simulink model "cic_dec3_poly_model"  (Simulink 7.4)
settings: Solver=ode45  StartTime=0.0  StopTime=10.0  RelTol=1e-3
libraries: xbsIndex_r4 x49
settings Model: Creator=chenhong  LastModifiedBy=chenhong

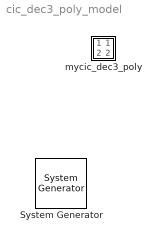
== system cic_dec3_poly_model ==
  " System Generator" : xbsIndex_r4/ System Generator  Tag=genX  SystemSampleTime=-1  xilinxfamily=Virtex6  part=xc6vsx315t  speed=-3  package=ff1156  synthesis_tool=XST  clock_wrapper=Clock Enables  directory=./netlist  testbench=off  simulink_period=1  sysclk_period=10  dcm_input_clock_period=10  incr_netlist=off  trim_vbits=Everywhere in SubSystem  dbl_ovrd=According to Block Masks  core_generation=According to Block Masks  run_coregen=off  deprecated_control=off  eval_field=0  block_type=sysgen
      settings: block_version=11.4
  mycic_dec3_poly : Subsystem

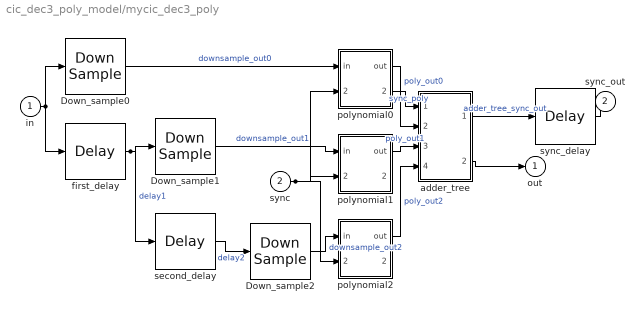
== system cic_dec3_poly_model/mycic_dec3_poly ==
  in : Inport
  sync : Inport  Port=2
  Down_sample0 : xbsIndex_r4/Down Sample  sample_ratio=3  sample_phase="Last Value of Frame  (most efficient)"  en=off  latency=1  dbl_ovrd=off  block_type=dsamp
      settings: block_version=11.4
  Down_sample1 : xbsIndex_r4/Down Sample  sample_ratio=3  sample_phase="Last Value of Frame  (most efficient)"  en=off  latency=1  dbl_ovrd=off  block_type=dsamp
      settings: block_version=11.4
  Down_sample2 : xbsIndex_r4/Down Sample  sample_ratio=3  sample_phase="Last Value of Frame  (most efficient)"  en=off  latency=1  dbl_ovrd=off  block_type=dsamp
      settings: block_version=11.4
  adder_tree : Subsystem
  first_delay : xbsIndex_r4/Delay  en=off  latency=1  dbl_ovrd=off  reg_retiming=off  block_type=delay
      settings: block_version=11.4
  polynomial0 : Subsystem
  polynomial1 : Subsystem
  polynomial2 : Subsystem
  second_delay : xbsIndex_r4/Delay  en=off  latency=1  dbl_ovrd=off  reg_retiming=off  block_type=delay
      settings: block_version=11.4
  sync_delay : xbsIndex_r4/Delay  en=off  latency=2  dbl_ovrd=off  reg_retiming=off  block_type=delay
      settings: block_version=11.4
  out : Outport
  sync_out : Outport  Port=2
  wires:
  in/1 -> first_delay/1, Down_sample0/1
  first_delay/1 -> second_delay/1, Down_sample1/1  "delay1"
  sync/1 -> polynomial2/2(sync), polynomial0/2(sync), polynomial1/2(sync)
  adder_tree/1(sync_out) -> sync_delay/1  "adder_tree_sync_out"
  adder_tree/2(dout) -> out/1
  polynomial1/1(out) -> adder_tree/3(din_2)  "poly_out1"
  polynomial0/2(sync_out) -> adder_tree/1(sync)  "sync_poly"
  Down_sample1/1 -> polynomial1/1(in)  "downsample_out1"
  second_delay/1 -> Down_sample2/1  "delay2"
  Down_sample0/1 -> polynomial0/1(in)  "downsample_out0"
  Down_sample2/1 -> polynomial2/1(in)  "downsample_out2"
  polynomial0/1(out) -> adder_tree/2(din_1)  "poly_out0"
  polynomial2/1(out) -> adder_tree/4(din_3)  "poly_out2"
  sync_delay/1 -> sync_out/1

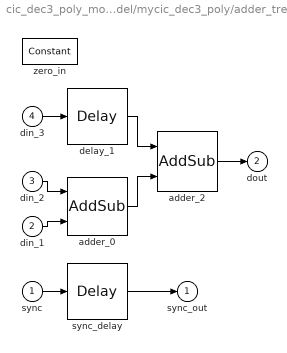
== system cic_dec3_poly_model/mycic_dec3_poly/adder_tree ==
  sync : Inport
  din_1 : Inport  Port=2
  din_2 : Inport  Port=3
  din_3 : Inport  Port=4
  adder_0 : xbsIndex_r4/AddSub  mode=Addition  use_carryin=off  use_carryout=off  en=off  latency=1  precision=Full  arith_type=Unsigned  n_bits=16  bin_pt=14  quantization="Round  (unbiased: +/- Inf)"  overflow=Saturate  dbl_ovrd=off  use_behavioral_HDL=on  hw_selection=Fabric  pipelined=off  block_type=addsub
  adder_2 : xbsIndex_r4/AddSub  mode=Addition  use_carryin=off  use_carryout=off  en=off  latency=1  precision=Full  arith_type=Unsigned  n_bits=16  bin_pt=14  quantization="Round  (unbiased: +/- Inf)"  overflow=Saturate  dbl_ovrd=off  use_behavioral_HDL=on  hw_selection=Fabric  pipelined=off  block_type=addsub
  delay_1 : xbsIndex_r4/Delay  en=off  latency=1  dbl_ovrd=off  reg_retiming=off  block_type=delay
      settings: block_version=11.4
  sync_delay : xbsIndex_r4/Delay  en=off  latency=2  dbl_ovrd=off  reg_retiming=off  block_type=delay
      settings: block_version=11.4
  zero_in : xbsIndex_r4/Constant  arith_type=Unsigned  const=0  n_bits=18  bin_pt=17  explicit_period=off  period=1  equ=P=C  opselect=C  inp2=PCIN>>17  opr=+  inp1=P  carry=CIN  dbl_ovrd=off  block_type=constant
      settings: block_version=11.4
  sync_out : Outport
  dout : Outport  Port=2
  wires:
  adder_0/1 -> adder_2/2
  din_2/1 -> adder_0/1
  sync/1 -> sync_delay/1
  sync_delay/1 -> sync_out/1
  din_1/1 -> adder_0/2
  din_3/1 -> delay_1/1
  delay_1/1 -> adder_2/1
  adder_2/1 -> dout/1

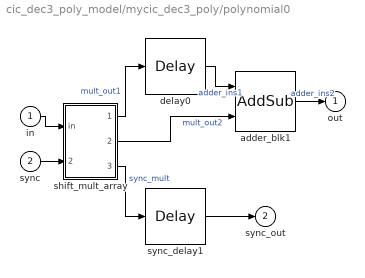
== system cic_dec3_poly_model/mycic_dec3_poly/polynomial0 ==
  in : Inport
  sync : Inport  Port=2
  adder_blk1 : xbsIndex_r4/AddSub  mode=Addition  use_carryin=off  use_carryout=off  en=off  latency=1  precision=Full  arith_type=Unsigned  n_bits=16  bin_pt=14  quantization=Truncate  overflow=Wrap  dbl_ovrd=off  use_behavioral_HDL=off  hw_selection=Fabric  pipelined=off  block_type=addsub
  delay0 : xbsIndex_r4/Delay  en=off  latency=1  dbl_ovrd=off  reg_retiming=off  block_type=delay
      settings: block_version=11.4
  shift_mult_array : Subsystem
  sync_delay1 : xbsIndex_r4/Delay  en=off  latency=1  dbl_ovrd=off  reg_retiming=off  block_type=delay
      settings: block_version=11.4
  out : Outport
  sync_out : Outport  Port=2
  wires:
  shift_mult_array/3(sync_out) -> sync_delay1/1  "sync_mult"
  delay0/1 -> adder_blk1/1  "adder_ins1"
  shift_mult_array/1(out1) -> delay0/1  "mult_out1"
  sync/1 -> shift_mult_array/2(sync)
  in/1 -> shift_mult_array/1(in)
  shift_mult_array/2(out2) -> adder_blk1/2  "mult_out2"
  adder_blk1/1 -> out/1  "adder_ins2"
  sync_delay1/1 -> sync_out/1

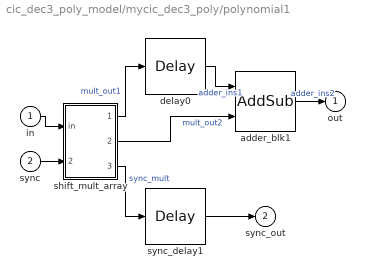
== system cic_dec3_poly_model/mycic_dec3_poly/polynomial1 ==
  in : Inport
  sync : Inport  Port=2
  adder_blk1 : xbsIndex_r4/AddSub  mode=Addition  use_carryin=off  use_carryout=off  en=off  latency=1  precision=Full  arith_type=Unsigned  n_bits=16  bin_pt=14  quantization=Truncate  overflow=Wrap  dbl_ovrd=off  use_behavioral_HDL=off  hw_selection=Fabric  pipelined=off  block_type=addsub
  delay0 : xbsIndex_r4/Delay  en=off  latency=1  dbl_ovrd=off  reg_retiming=off  block_type=delay
      settings: block_version=11.4
  shift_mult_array : Subsystem
  sync_delay1 : xbsIndex_r4/Delay  en=off  latency=1  dbl_ovrd=off  reg_retiming=off  block_type=delay
      settings: block_version=11.4
  out : Outport
  sync_out : Outport  Port=2
  wires:
  shift_mult_array/3(sync_out) -> sync_delay1/1  "sync_mult"
  delay0/1 -> adder_blk1/1  "adder_ins1"
  shift_mult_array/1(out1) -> delay0/1  "mult_out1"
  sync/1 -> shift_mult_array/2(sync)
  in/1 -> shift_mult_array/1(in)
  shift_mult_array/2(out2) -> adder_blk1/2  "mult_out2"
  adder_blk1/1 -> out/1  "adder_ins2"
  sync_delay1/1 -> sync_out/1

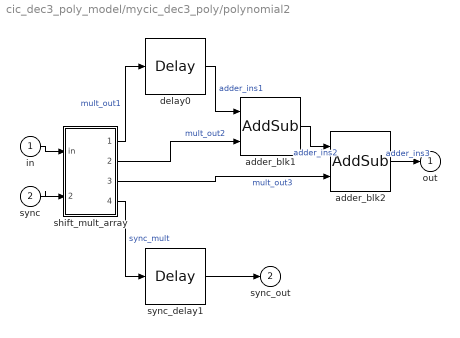
== system cic_dec3_poly_model/mycic_dec3_poly/polynomial2 ==
  in : Inport
  sync : Inport  Port=2
  adder_blk1 : xbsIndex_r4/AddSub  mode=Addition  use_carryin=off  use_carryout=off  en=off  latency=1  precision=Full  arith_type=Unsigned  n_bits=16  bin_pt=14  quantization=Truncate  overflow=Wrap  dbl_ovrd=off  use_behavioral_HDL=off  hw_selection=Fabric  pipelined=off  block_type=addsub
  adder_blk2 : xbsIndex_r4/AddSub  mode=Addition  use_carryin=off  use_carryout=off  en=off  latency=1  precision=Full  arith_type=Unsigned  n_bits=16  bin_pt=14  quantization=Truncate  overflow=Wrap  dbl_ovrd=off  use_behavioral_HDL=off  hw_selection=Fabric  pipelined=off  block_type=addsub
  delay0 : xbsIndex_r4/Delay  en=off  latency=1  dbl_ovrd=off  reg_retiming=off  block_type=delay
      settings: block_version=11.4
  shift_mult_array : Subsystem
  sync_delay1 : xbsIndex_r4/Delay  en=off  latency=1  dbl_ovrd=off  reg_retiming=off  block_type=delay
      settings: block_version=11.4
  out : Outport
  sync_out : Outport  Port=2
  wires:
  shift_mult_array/4(sync_out) -> sync_delay1/1  "sync_mult"
  adder_blk1/1 -> adder_blk2/1  "adder_ins2"
  shift_mult_array/2(out2) -> adder_blk1/2  "mult_out2"
  in/1 -> shift_mult_array/1(in)
  sync/1 -> shift_mult_array/2(sync)
  shift_mult_array/1(out1) -> delay0/1  "mult_out1"
  delay0/1 -> adder_blk1/1  "adder_ins1"
  shift_mult_array/3(out3) -> adder_blk2/2  "mult_out3"
  adder_blk2/1 -> out/1  "adder_ins3"
  sync_delay1/1 -> sync_out/1

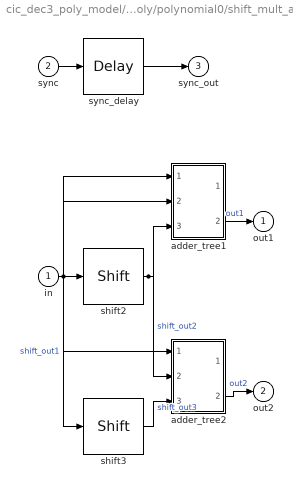
== system cic_dec3_poly_model/mycic_dec3_poly/polynomial0/shift_mult_array ==
  in : Inport
  sync : Inport  Port=2
  adder_tree1 : Subsystem
  adder_tree2 : Subsystem
  shift2 : xbsIndex_r4/Shift  shift_dir=Left  shift_bits=1  en=off  latency=0  precision=User Defined  arith_type="Signed  (2's comp)"  n_bits=9  bin_pt=3  quantization=Truncate  overflow=Wrap  dbl_ovrd=off  block_type=shift
  shift3 : xbsIndex_r4/Shift  shift_dir=Left  shift_bits=2  en=off  latency=0  precision=User Defined  arith_type="Signed  (2's comp)"  n_bits=10  bin_pt=3  quantization=Truncate  overflow=Wrap  dbl_ovrd=off  block_type=shift
  sync_delay : xbsIndex_r4/Delay  en=off  latency=1  dbl_ovrd=off  reg_retiming=off  block_type=delay
      settings: block_version=11.4
  out1 : Outport
  out2 : Outport  Port=2
  sync_out : Outport  Port=3
  wires:
  in/1 -> adder_tree2/1(sync), adder_tree1/1(sync), shift3/1, shift2/1, adder_tree1/2(din_1)  "shift_out1"
  shift2/1 -> adder_tree1/3(din_2), adder_tree2/2(din_1)  "shift_out2"
  sync/1 -> sync_delay/1
  adder_tree1/2(dout) -> out1/1  "out1"
  shift3/1 -> adder_tree2/3(din_2)  "shift_out3"
  adder_tree2/2(dout) -> out2/1  "out2"
  sync_delay/1 -> sync_out/1

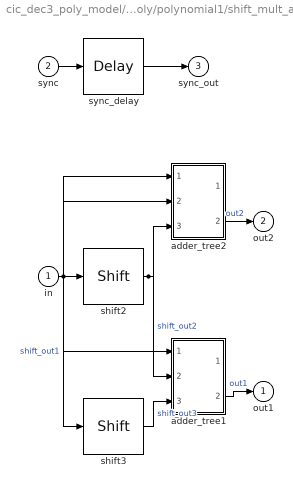
== system cic_dec3_poly_model/mycic_dec3_poly/polynomial1/shift_mult_array ==
  in : Inport
  sync : Inport  Port=2
  adder_tree1 : Subsystem
  adder_tree2 : Subsystem
  shift2 : xbsIndex_r4/Shift  shift_dir=Left  shift_bits=1  en=off  latency=0  precision=User Defined  arith_type="Signed  (2's comp)"  n_bits=9  bin_pt=3  quantization=Truncate  overflow=Wrap  dbl_ovrd=off  block_type=shift
  shift3 : xbsIndex_r4/Shift  shift_dir=Left  shift_bits=2  en=off  latency=0  precision=User Defined  arith_type="Signed  (2's comp)"  n_bits=10  bin_pt=3  quantization=Truncate  overflow=Wrap  dbl_ovrd=off  block_type=shift
  sync_delay : xbsIndex_r4/Delay  en=off  latency=1  dbl_ovrd=off  reg_retiming=off  block_type=delay
      settings: block_version=11.4
  out1 : Outport
  out2 : Outport  Port=2
  sync_out : Outport  Port=3
  wires:
  in/1 -> adder_tree2/1(sync), adder_tree1/1(sync), shift3/1, shift2/1, adder_tree2/2(din_1)  "shift_out1"
  shift2/1 -> adder_tree2/3(din_2), adder_tree1/2(din_1)  "shift_out2"
  sync/1 -> sync_delay/1
  adder_tree1/2(dout) -> out1/1  "out1"
  shift3/1 -> adder_tree1/3(din_2)  "shift_out3"
  adder_tree2/2(dout) -> out2/1  "out2"
  sync_delay/1 -> sync_out/1

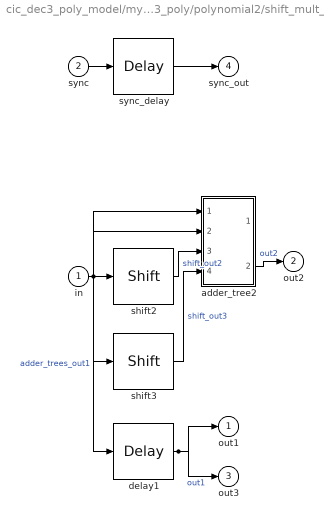
== system cic_dec3_poly_model/mycic_dec3_poly/polynomial2/shift_mult_array ==
  in : Inport
  sync : Inport  Port=2
  adder_tree2 : Subsystem
  delay1 : xbsIndex_r4/Delay  en=off  latency=2  dbl_ovrd=off  reg_retiming=off  block_type=delay
      settings: block_version=11.4
  shift2 : xbsIndex_r4/Shift  shift_dir=Left  shift_bits=1  en=off  latency=0  precision=User Defined  arith_type="Signed  (2's comp)"  n_bits=9  bin_pt=3  quantization=Truncate  overflow=Wrap  dbl_ovrd=off  block_type=shift
  shift3 : xbsIndex_r4/Shift  shift_dir=Left  shift_bits=2  en=off  latency=0  precision=User Defined  arith_type="Signed  (2's comp)"  n_bits=10  bin_pt=3  quantization=Truncate  overflow=Wrap  dbl_ovrd=off  block_type=shift
  sync_delay : xbsIndex_r4/Delay  en=off  latency=2  dbl_ovrd=off  reg_retiming=off  block_type=delay
      settings: block_version=11.4
  out1 : Outport
  out2 : Outport  Port=2
  out3 : Outport  Port=3
  sync_out : Outport  Port=4
  wires:
  in/1 -> adder_tree2/1(sync), shift3/1, shift2/1, adder_tree2/2(din_1), delay1/1  "adder_trees_out1"
  delay1/1 -> out1/1, out3/1  "out1"
  sync/1 -> sync_delay/1
  adder_tree2/2(dout) -> out2/1  "out2"
  shift2/1 -> adder_tree2/3(din_2)  "shift_out2"
  shift3/1 -> adder_tree2/4(din_3)  "shift_out3"
  sync_delay/1 -> sync_out/1

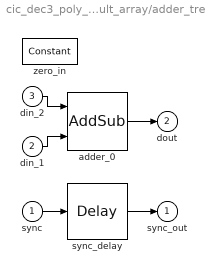
== system cic_dec3_poly_model/mycic_dec3_poly/polynomial0/shift_mult_array/adder_tree1 ==
  sync : Inport
  din_1 : Inport  Port=2
  din_2 : Inport  Port=3
  adder_0 : xbsIndex_r4/AddSub  mode=Addition  use_carryin=off  use_carryout=off  en=off  latency=1  precision=Full  arith_type=Unsigned  n_bits=16  bin_pt=14  quantization="Round  (unbiased: +/- Inf)"  overflow=Saturate  dbl_ovrd=off  use_behavioral_HDL=on  hw_selection=Fabric  pipelined=off  block_type=addsub
  sync_delay : xbsIndex_r4/Delay  en=off  latency=1  dbl_ovrd=off  reg_retiming=off  block_type=delay
      settings: block_version=11.4
  zero_in : xbsIndex_r4/Constant  arith_type=Unsigned  const=0  n_bits=18  bin_pt=17  explicit_period=off  period=1  equ=P=C  opselect=C  inp2=PCIN>>17  opr=+  inp1=P  carry=CIN  dbl_ovrd=off  block_type=constant
      settings: block_version=11.4
  sync_out : Outport
  dout : Outport  Port=2
  wires:
  din_1/1 -> adder_0/2
  sync_delay/1 -> sync_out/1
  sync/1 -> sync_delay/1
  din_2/1 -> adder_0/1
  adder_0/1 -> dout/1

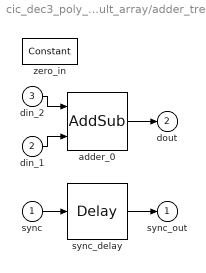
== system cic_dec3_poly_model/mycic_dec3_poly/polynomial0/shift_mult_array/adder_tree2 ==
  sync : Inport
  din_1 : Inport  Port=2
  din_2 : Inport  Port=3
  adder_0 : xbsIndex_r4/AddSub  mode=Addition  use_carryin=off  use_carryout=off  en=off  latency=1  precision=Full  arith_type=Unsigned  n_bits=16  bin_pt=14  quantization="Round  (unbiased: +/- Inf)"  overflow=Saturate  dbl_ovrd=off  use_behavioral_HDL=on  hw_selection=Fabric  pipelined=off  block_type=addsub
  sync_delay : xbsIndex_r4/Delay  en=off  latency=1  dbl_ovrd=off  reg_retiming=off  block_type=delay
      settings: block_version=11.4
  zero_in : xbsIndex_r4/Constant  arith_type=Unsigned  const=0  n_bits=18  bin_pt=17  explicit_period=off  period=1  equ=P=C  opselect=C  inp2=PCIN>>17  opr=+  inp1=P  carry=CIN  dbl_ovrd=off  block_type=constant
      settings: block_version=11.4
  sync_out : Outport
  dout : Outport  Port=2
  wires:
  din_1/1 -> adder_0/2
  sync_delay/1 -> sync_out/1
  sync/1 -> sync_delay/1
  din_2/1 -> adder_0/1
  adder_0/1 -> dout/1

== system cic_dec3_poly_model/mycic_dec3_poly/polynomial1/shift_mult_array/adder_tree1 ==
  sync : Inport
  din_1 : Inport  Port=2
  din_2 : Inport  Port=3
  adder_0 : xbsIndex_r4/AddSub  mode=Addition  use_carryin=off  use_carryout=off  en=off  latency=1  precision=Full  arith_type=Unsigned  n_bits=16  bin_pt=14  quantization="Round  (unbiased: +/- Inf)"  overflow=Saturate  dbl_ovrd=off  use_behavioral_HDL=on  hw_selection=Fabric  pipelined=off  block_type=addsub
  sync_delay : xbsIndex_r4/Delay  en=off  latency=1  dbl_ovrd=off  reg_retiming=off  block_type=delay
      settings: block_version=11.4
  zero_in : xbsIndex_r4/Constant  arith_type=Unsigned  const=0  n_bits=18  bin_pt=17  explicit_period=off  period=1  equ=P=C  opselect=C  inp2=PCIN>>17  opr=+  inp1=P  carry=CIN  dbl_ovrd=off  block_type=constant
      settings: block_version=11.4
  sync_out : Outport
  dout : Outport  Port=2
  wires:
  din_1/1 -> adder_0/2
  sync_delay/1 -> sync_out/1
  sync/1 -> sync_delay/1
  din_2/1 -> adder_0/1
  adder_0/1 -> dout/1

== system cic_dec3_poly_model/mycic_dec3_poly/polynomial1/shift_mult_array/adder_tree2 ==
  sync : Inport
  din_1 : Inport  Port=2
  din_2 : Inport  Port=3
  adder_0 : xbsIndex_r4/AddSub  mode=Addition  use_carryin=off  use_carryout=off  en=off  latency=1  precision=Full  arith_type=Unsigned  n_bits=16  bin_pt=14  quantization="Round  (unbiased: +/- Inf)"  overflow=Saturate  dbl_ovrd=off  use_behavioral_HDL=on  hw_selection=Fabric  pipelined=off  block_type=addsub
  sync_delay : xbsIndex_r4/Delay  en=off  latency=1  dbl_ovrd=off  reg_retiming=off  block_type=delay
      settings: block_version=11.4
  zero_in : xbsIndex_r4/Constant  arith_type=Unsigned  const=0  n_bits=18  bin_pt=17  explicit_period=off  period=1  equ=P=C  opselect=C  inp2=PCIN>>17  opr=+  inp1=P  carry=CIN  dbl_ovrd=off  block_type=constant
      settings: block_version=11.4
  sync_out : Outport
  dout : Outport  Port=2
  wires:
  din_1/1 -> adder_0/2
  sync_delay/1 -> sync_out/1
  sync/1 -> sync_delay/1
  din_2/1 -> adder_0/1
  adder_0/1 -> dout/1

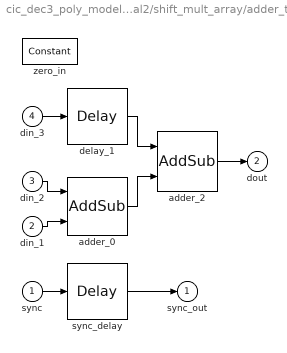
== system cic_dec3_poly_model/mycic_dec3_poly/polynomial2/shift_mult_array/adder_tree2 ==
  sync : Inport
  din_1 : Inport  Port=2
  din_2 : Inport  Port=3
  din_3 : Inport  Port=4
  adder_0 : xbsIndex_r4/AddSub  mode=Addition  use_carryin=off  use_carryout=off  en=off  latency=1  precision=Full  arith_type=Unsigned  n_bits=16  bin_pt=14  quantization="Round  (unbiased: +/- Inf)"  overflow=Saturate  dbl_ovrd=off  use_behavioral_HDL=on  hw_selection=Fabric  pipelined=off  block_type=addsub
  adder_2 : xbsIndex_r4/AddSub  mode=Addition  use_carryin=off  use_carryout=off  en=off  latency=1  precision=Full  arith_type=Unsigned  n_bits=16  bin_pt=14  quantization="Round  (unbiased: +/- Inf)"  overflow=Saturate  dbl_ovrd=off  use_behavioral_HDL=on  hw_selection=Fabric  pipelined=off  block_type=addsub
  delay_1 : xbsIndex_r4/Delay  en=off  latency=1  dbl_ovrd=off  reg_retiming=off  block_type=delay
      settings: block_version=11.4
  sync_delay : xbsIndex_r4/Delay  en=off  latency=2  dbl_ovrd=off  reg_retiming=off  block_type=delay
      settings: block_version=11.4
  zero_in : xbsIndex_r4/Constant  arith_type=Unsigned  const=0  n_bits=18  bin_pt=17  explicit_period=off  period=1  equ=P=C  opselect=C  inp2=PCIN>>17  opr=+  inp1=P  carry=CIN  dbl_ovrd=off  block_type=constant
      settings: block_version=11.4
  sync_out : Outport
  dout : Outport  Port=2
  wires:
  adder_0/1 -> adder_2/2
  din_2/1 -> adder_0/1
  sync/1 -> sync_delay/1
  sync_delay/1 -> sync_out/1
  din_1/1 -> adder_0/2
  din_3/1 -> delay_1/1
  delay_1/1 -> adder_2/1
  adder_2/1 -> dout/1
